simulink model "threephasefullycontrolledconverter"  (R2023b)
settings: Solver=VariableStepAuto  StartTime=0.0  StopTime=0.5  RelTol=1e-3
libraries: spsDetailedThyristorLib x6, spsTHDLib x4, spsACVoltageSourceLib x3, spsRMSLib x2, spsSeriesRLCBranchLib x2, spsCurrentMeasurementLib x1, spsDCVoltageSourceLib x1, spsDiodeLib x1, spsGroundLib x1, spsThreePhaseVIMeasurementLib x1, spsVoltageMeasurementLib x1, sps_lib x1
settings Model: Creator=Anusha  LastModifiedBy=Anusha

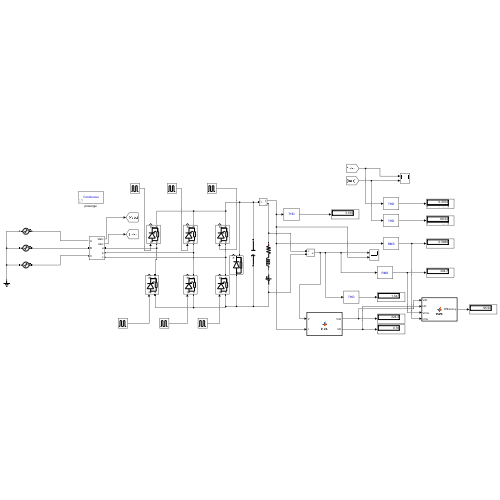
[thumbnail: Simulink's stored preview of the top-level diagram]
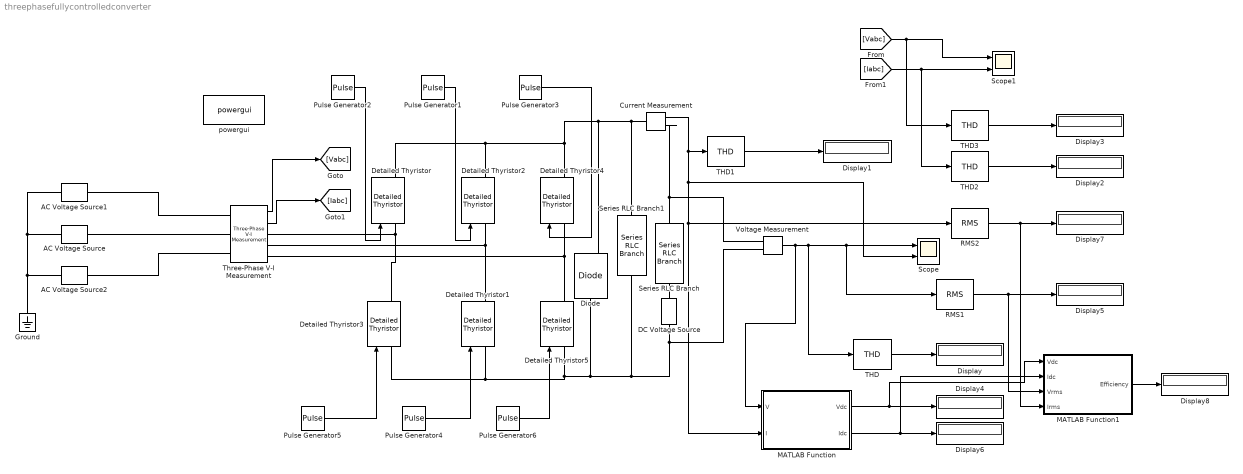
== system threephasefullycontrolledconverter ==
  AC Voltage Source : spsACVoltageSourceLib/AC Voltage Source  Amplitude=230  Phase=120  Frequency=50  SampleTime=0  Measurements=None  BusType=swing  Pref=10e3  Qref=0  Qmin=-inf  Qmax=+inf
  AC Voltage Source1 : spsACVoltageSourceLib/AC Voltage Source  Amplitude=230  Phase=0  Frequency=50  SampleTime=0  Measurements=None  BusType=swing  Pref=10e3  Qref=0  Qmin=-inf  Qmax=+inf
  AC Voltage Source2 : spsACVoltageSourceLib/AC Voltage Source  Amplitude=230  Phase=240  Frequency=50  SampleTime=0  Measurements=None  BusType=swing  Pref=10e3  Qref=0  Qmin=-inf  Qmax=+inf
  Current Measurement : spsCurrentMeasurementLib/Current Measurement  PhasorSimulation=off  OutputType=Complex  PSBequivalent=0
  DC Voltage Source : spsDCVoltageSourceLib/DC Voltage Source  Amplitude=200  Measurements=None
  Detailed Thyristor{,1..5} (6 alike) : spsDetailedThyristorLib/Detailed Thyristor  Ron=0.001  Lon=1e-3  Vf=0.8  IL=0.1  Tq=100e-6  IC=0  Rs=500  Cs=250e-9  Measurements=on
      settings: LibrarySourceBlock=sps_lib/Power Electronics/Detailed Thyristor
  Diode : spsDiodeLib/Diode  Ron=0.001  Lon=0  Vf=0.8  IC=0  UseSnubber=0  Rs=500  Cs=250e-9  Measurements=on
  Display{,1..8} (9 alike) : Display
  Ground : spsGroundLib/Ground  LConnTagsString=a
  MATLAB Function : MATLAB Function  TreatAsAtomicUnit=on
  MATLAB Function1 : MATLAB Function  TreatAsAtomicUnit=on
  Pulse Generator1 : DiscretePulseGenerator  PulseType=Time based  Period=0.02  PulseWidth=33.35  PhaseDelay=0.01
  Pulse Generator2 : DiscretePulseGenerator  PulseType=Time based  Period=0.02  PulseWidth=33.35  PhaseDelay=0.0033
  Pulse Generator3 : DiscretePulseGenerator  PulseType=Time based  Period=0.02  PulseWidth=33.35  PhaseDelay=0.01663
  Pulse Generator4 : DiscretePulseGenerator  PulseType=Time based  Period=0.02  PulseWidth=33.35  PhaseDelay=0.02
  Pulse Generator5 : DiscretePulseGenerator  PulseType=Time based  Period=0.02  PulseWidth=33.35  PhaseDelay=0.01333
  Pulse Generator6 : DiscretePulseGenerator  PulseType=Time based  Period=0.02  PulseWidth=33.35  PhaseDelay=0.00663
  RMS1 : spsRMSLib/RMS  TrueRMS=on  Freq=60  RMSInit=120  Ts=0
  RMS2 : spsRMSLib/RMS  TrueRMS=on  Freq=60  RMSInit=120  Ts=0
  Scope : Scope  NumInputPorts=2
  Scope1 : Scope  NumInputPorts=2
  Series RLC Branch : spsSeriesRLCBranchLib/Series RLC Branch  LConnTagsString=__new0  RConnTagsString=__new0  BranchType=RL  Resistance=100  Inductance=1  SetiL0=off  InitialCurrent=0  Capacitance=1e-6  Setx0=off  InitialVoltage=0  Measurements=None
  Series RLC Branch1 : spsSeriesRLCBranchLib/Series RLC Branch  LConnTagsString=__new0  RConnTagsString=__new0  BranchType=C  Resistance=100  Inductance=1  SetiL0=off  InitialCurrent=0  Capacitance=1e-5  Setx0=off  InitialVoltage=0  Measurements=None
  THD{,1..3} (4 alike) : spsTHDLib/THD  Freq=60  Ts=0
  Three-Phase V-I Measurement : spsThreePhaseVIMeasurementLib/Three-Phase V-I Measurement  VoltageMeasurement=phase-to-phase  SetLabelV=off  LabelV=Vabc  Vpu=off  VpuLL=off  CurrentMeasurement=yes  SetLabelI=off  LabelI=Iabc  Ipu=off  Pbase=100e6  Vbase=500e3  OutputType=Complex  PhasorSimulation=off  PSBequivalent=0
  Voltage Measurement : spsVoltageMeasurementLib/Voltage Measurement  PhasorSimulation=off  OutputType=Complex  PSBequivalent=0
  powergui : sps_lib/powergui  Priority=1  SimulationMode=Continuous  SampleTime=50e-6  frequency=60  Iterations=50  frequencyindice=50  Pbase=100e6  ErrMax=1e-4  UnitsV=kV  UnitsW=MW  buscounter=0  FunctionMessages=off  echomessages=off  EnableUseOfTLC=off  CurrentSourceSwitches=off  DisableSnubberDevices=off  DisableRonSwitches=off  DisableVfSwitches=off  DisplayEquations=off  AutomaticDiscreteSolvers=off  SolverType=Tustin/Backward Euler (TBE)  Interpol=off  ExternalGateDelay=off  methode=off  Ts=100  x0status=blocks  SPID=on  SwTol=0  HookPort=off  NonlinearTolerance=1e-4  nMaxIteration=100  ContinueOnMaxIteration=off  RestoreLinks=warning  ResistiveCurrentMeasurement=off  Frange=[0:2:500]  Ylog=off  Xlog=on  ShowGrid=off  save=off  variable=ZData  structure=0  ZoomFFT=off  StartTime=0.0  cycles=1  DisplayStyle=1  fundamental=60  FreqAxis=off  MaxFrequency=1000  frequencyindicesteady=1  RmsSteady=1  display=off
  wires:
  THD/1 -> Display/1
  Pulse Generator2/1 -> Detailed Thyristor/1
  Pulse Generator1/1 -> Detailed Thyristor2/1
  Pulse Generator3/1 -> Detailed Thyristor4/1
  Pulse Generator5/1 -> Detailed Thyristor3/1
  Pulse Generator4/1 -> Detailed Thyristor1/1
  Pulse Generator6/1 -> Detailed Thyristor5/1
  Three-Phase V-I Measurement/1 -> [Vabc]
  Three-Phase V-I Measurement/2 -> [Iabc]
  [Vabc] -> THD3/1, Scope1/1
  [Iabc] -> THD2/1, Scope1/2
  THD1/1 -> Display1/1
  THD2/1 -> Display2/1
  THD3/1 -> Display3/1
  Voltage Measurement/1 -> MATLAB Function/1(V), THD/1, RMS1/1, Scope/1
  RMS1/1 -> MATLAB Function1/3(Vrms), Display5/1
  Current Measurement/1 -> RMS2/1, MATLAB Function/2(I), Scope/2, THD1/1
  MATLAB Function/1(Vdc) -> MATLAB Function1/1(Vdc), Display4/1
  MATLAB Function/2(Idc) -> MATLAB Function1/2(Idc), Display6/1
  RMS2/1 -> Display7/1, MATLAB Function1/4(Irms)
  MATLAB Function1/1(Efficiency) -> Display8/1
  connections:
  Detailed Thyristor/LConn1 -- Three-Phase V-I Measurement/RConn1 -- Detailed Thyristor3/RConn1
  Detailed Thyristor1/RConn1 -- Three-Phase V-I Measurement/RConn2 -- Detailed Thyristor2/LConn1
  Detailed Thyristor5/RConn1 -- Three-Phase V-I Measurement/RConn3 -- Detailed Thyristor4/LConn1
  Detailed Thyristor/RConn1 -- Detailed Thyristor2/RConn1 -- Series RLC Branch1/LConn1 -- Current Measurement/LConn1 -- Diode/RConn1 -- Detailed Thyristor4/RConn1
  Detailed Thyristor3/LConn1 -- Detailed Thyristor1/LConn1 -- DC Voltage Source/LConn1 -- Voltage Measurement/LConn2 -- Series RLC Branch1/RConn1 -- Diode/LConn1 -- Detailed Thyristor5/LConn1
  Series RLC Branch/LConn1 -- Current Measurement/RConn1 -- Voltage Measurement/LConn1
  Three-Phase V-I Measurement/LConn1 -- AC Voltage Source1/RConn1
  Three-Phase V-I Measurement/LConn2 -- AC Voltage Source/RConn1
  Three-Phase V-I Measurement/LConn3 -- AC Voltage Source2/RConn1
  AC Voltage Source2/LConn1 -- AC Voltage Source/LConn1 -- AC Voltage Source1/LConn1 -- Ground/LConn1
  DC Voltage Source/RConn1 -- Series RLC Branch/RConn1

== matlab function threephasefullycontrolledconverter/MATLAB Function1 ==
  data: Vdc input; Efficiency output; Idc input; Vrms input; Irms input
function Efficiency   = stats(Vdc,Idc,Vrms,Irms)

Efficiency=((Vdc*Idc)/(Vrms*Irms))*100;

== matlab function threephasefullycontrolledconverter/MATLAB Function ==
  data: V input; Vdc output; I input; Idc output
function [Vdc,Idc]  = stats(V,I)

Vdc=mean(V);
Idc=mean(I);
